simulink subsystem "testSubject"  (R2023a)
settings: Solver=VariableStepAuto  StartTime=0.0  StopTime=10.0  RelTol=1e-3
libraries: simulink x2
settings Model: Creator=diontep  LastModifiedBy=diontep

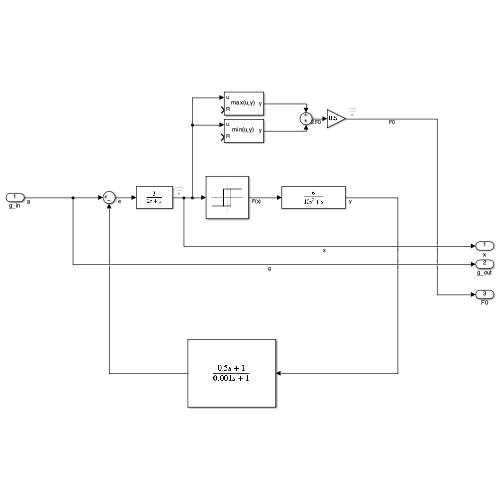
[thumbnail: Simulink's stored preview of the top-level diagram]
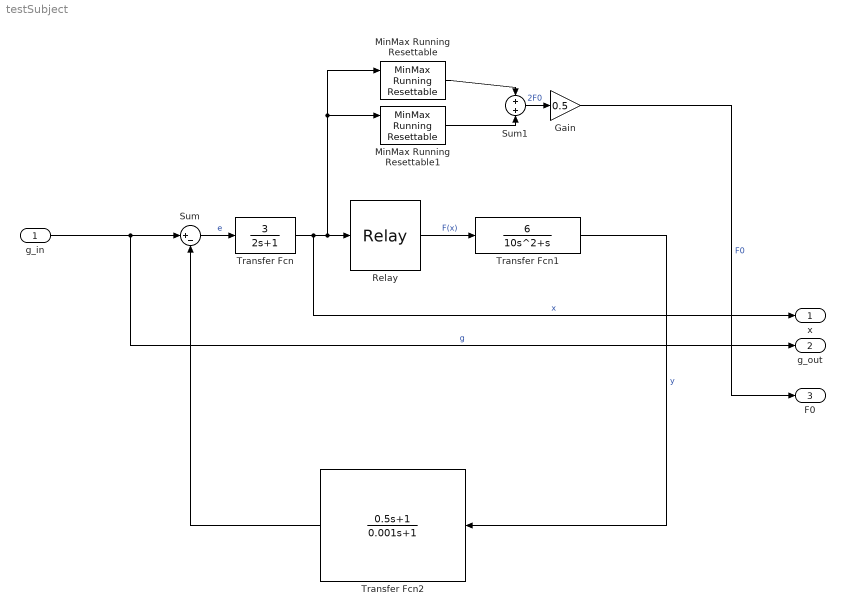
== system testSubject ==
  g_in : Inport
  Gain : Gain  Gain=0.5
  MinMax Running Resettable : simulink/Math Operations/MinMax Running Resettable  Function=max  vinit=0.0
  MinMax Running Resettable1 : simulink/Math Operations/MinMax Running Resettable  Function=min  vinit=0.0
  Relay : Relay  OnSwitchValue=0  OffSwitchValue=0  OnOutputValue=pi/2  OffOutputValue=-pi/2
  Sum : Sum  Inputs=|+-
  Sum1 : Sum
  Transfer Fcn : TransferFcn  Numerator=[3]  Denominator=[2 1]
  Transfer Fcn1 : TransferFcn  Numerator=[6]  Denominator=[10 1 0]
  Transfer Fcn2 : TransferFcn  Numerator=[0.5 1]  Denominator=[0.001 1]
  x : Outport
  g_out : Outport  Port=2
  F0 : Outport  Port=3
  wires:
  g_in/1 -> g_out/1, Sum/1  "g"
  Transfer Fcn1/1 -> Transfer Fcn2/1  "y"
  MinMax Running Resettable/1 -> Sum1/1
  Transfer Fcn/1 -> x/1, MinMax Running Resettable1/1, MinMax Running Resettable/1, Relay/1  "x"
  Relay/1 -> Transfer Fcn1/1  "F(x)"
  Gain/1 -> F0/1  "F0"
  Sum1/1 -> Gain/1  "2F0"
  Transfer Fcn2/1 -> Sum/2
  Sum/1 -> Transfer Fcn/1  "e"
  MinMax Running Resettable1/1 -> Sum1/2
